simulink model "W08_F_mission"  (R2024b)
settings: Solver=ode4  StartTime=0  StopTime=T_final  FixedStep=h  RelTol=1e-3
values from neighbouring files (symbols this model uses):
  beta_c = pi/2    (= 1.57079632679)    [W08_0_setup.m]
  Delta = 5    [W08_0_setup.m]
  E_hold = 0    [W08_0_setup.m]
  e_min = 0.3    [W08_0_setup.m]
  h = 0.02    [W08_0_setup.m]    (also in W08_1_build_dp.m = add_line(sys, [a; via; b]))
  hand_over = 1    [W08_0_setup.m]
  k_neg = cfg.k_neg    [W08_0_setup.m]
  k_pos = cfg.k_pos    [W08_0_setup.m]
  Kd = 100    [W08_0_setup.m]
  Kd_x = 60    [W08_0_setup.m]
  Ki_x = 3    [W08_0_setup.m]
  Kp = 300    [W08_0_setup.m]
  Kp_x = 30    [W08_0_setup.m]
  mp = 25    [W08_0_setup.m]
  N_hold = 0    [W08_0_setup.m]
  N_max = min(2*cfg.y_pont*(cfg.k_pos*cfg.n_max^2 - X_max/2),              2*cfg.y_pont*(X_max/2 + cfg.k_neg*cfg.n_min^2))    [W08_0_setup.m]
  R_arrive = 2    [W08_0_setup.m]
  rp = [0.05 0 -0.35]'    [W08_0_setup.m]
  T_hold = 40    [W08_0_setup.m]
  T_max = cfg.k_pos*cfg.n_max^2    [W08_0_setup.m]
  T_min = -cfg.k_neg*cfg.n_min^2    [W08_0_setup.m]
  V_c = 0.3    [W08_0_setup.m]
  WP_E = [0  0 40]'    [W08_0_setup.m]
  WP_N = [0 40 40]'    [W08_0_setup.m]
  x0 = zeros(12,1)    [W08_0_setup.m]    (also in W08_E_cascade_gains.m = zeros(12,1);  x0(8) = 5)
  X_ff = 60    [W08_0_setup.m]
  X_max = 120    [W08_0_setup.m]
  y_pont = cfg.y_pont    [W08_0_setup.m]
settings Model: Creator=admin  LastModifiedBy=admin
settings DataIOCC: ReturnWorkspaceOutputs=off

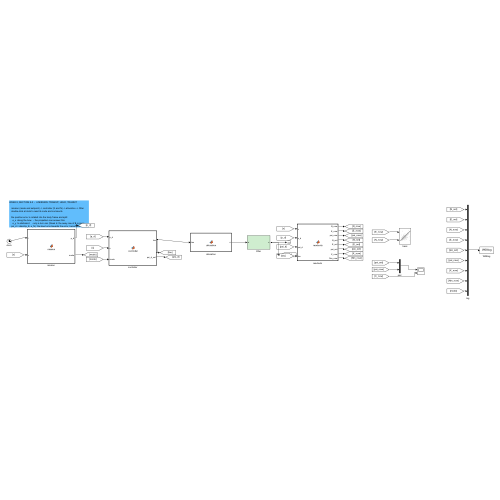
[thumbnail: Simulink's stored preview of the top-level diagram]
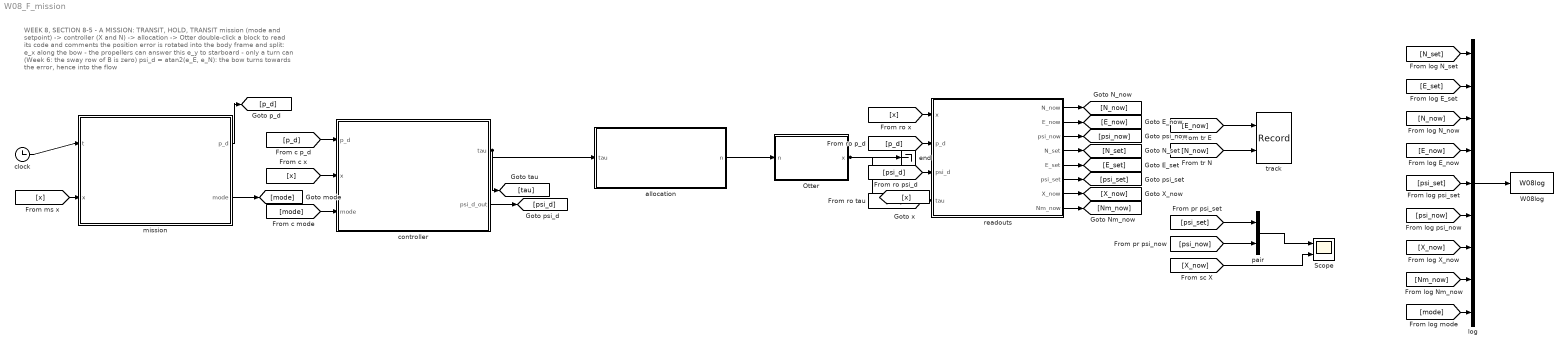
== system W08_F_mission ==
  note: WEEK 8, SECTION 8-5  -  A MISSION: TRANSIT, HOLD, TRANSIT
      |
      |    mission (mode and setpoint) -> controller (X and N) -> allocation -> Otter
      |    double-click a block to read its code and comments
      |
      |    the position error is rotated into the body frame and split:
      |      e_x  along the bow   - the propellers can answer this
      |      e_y  to starboard    - only a turn can (Week 6: the sway row of B is zero)
      |    psi_d = atan2(e_E, e_N): the bow turns towards the error, hence into the flow
  Otter : Subsystem
  Scope : Scope  NumInputPorts=2
  W08log : ToWorkspace  VariableName=W08log  SaveFormat=Structure With Time  SampleTime=-1
  allocation : MATLAB Function  TreatAsAtomicUnit=on
  clock : Clock
  controller : MATLAB Function  TreatAsAtomicUnit=on
  end : Terminator
  log : Mux  Inputs=9
  mission : MATLAB Function  TreatAsAtomicUnit=on
  pair : Mux  Inputs=2
  readouts : MATLAB Function  TreatAsAtomicUnit=on
  track : Record  FileSettingsInternal="{\"entries\":[{\"content\":{\"excelSettings\":{\"content\":{},\"type\":\"Streamout.ExcelSettings\"}},\"type\":\"Streamout.FileSettingStorage\",\"uuid\":\"\"}],\"packageUris\":[\"http:\\/\\/schema.mathworks.com\\/mf0\\/streamout_blocks\\/R2020a\"],\"version\":\"1.0\"}"  Layout=[1 1]  SignalsInternal="{\"entries\":[{\"content\":{\"signals\":[{\"content\":{\"blockPath\":[],\"dimensions\":[1],\"domain\":\"\",\"lineColor\":\"#a2142f\",\"plots\":[ 1 ],\"port\":1,\"signalID\":1,\"signalName\":\"XY Graph:1\"},\"type\":\"RecordBlkView.Signal\",\"uuid\":\"\"},{\"content\":{\"blockPath\":[],\"dimensions\":[1],\"domain\":\"\",\"lineColor\":\"#139fff\",\"plots\":[ 1 ],\"port\":2,\"signalID\":2,\"signalName\":\"XY Graph:2\"},\"type\":\"RecordBlkView.Signal\",\"uuid\":\"\"}]},\"type\":\"RecordBlkView.InputSignals\",\"uuid\":\"\"}],\"packageUris\":[\"http:\\/\\/schema.mathworks.com\\/mf0\\/streamout_blocks\\/R2020a\"],\"version\":\"1.0\"}"  VisualizationBindings="{\"xyplotplugin\":{\"info\":[{\"series\":[{\"bindingParametersList\":[{\"parameter\":\"X-Axis\",\"signalID\":1,\"signalName\":\"XY Graph:1\"},{\"parameter\":\"Y-Axis\",\"signalID\":2,\"signalName\":\"XY Graph:2\"}],\"seriesID\":0}],\"subplotID\":1}]}}"  CompatibilityTag=XY
  wires:
  clock/1 -> mission/1(t)
  [x] -> mission/2(x)
  mission/1(p_d) -> [p_d]
  mission/2(mode) -> [mode]
  [p_d] -> controller/1(p_d)
  [x] -> controller/2(x)
  [mode] -> controller/3(mode)
  controller/1(tau) -> [tau], allocation/1(tau)
  controller/2(psi_d_out) -> [psi_d]
  allocation/1(n) -> Otter/1(n)
  Otter/1(x) -> [x], end/1
  [x] -> readouts/1(x)
  [p_d] -> readouts/2(p_d)
  [psi_d] -> readouts/3(psi_d)
  [tau] -> readouts/4(tau)
  readouts/1(N_now) -> [N_now]
  readouts/2(E_now) -> [E_now]
  readouts/3(psi_now) -> [psi_now]
  readouts/4(N_set) -> [N_set]
  readouts/5(E_set) -> [E_set]
  readouts/6(psi_set) -> [psi_set]
  readouts/7(X_now) -> [X_now]
  readouts/8(Nm_now) -> [Nm_now]
  [E_now] -> track/1
  [N_now] -> track/2
  [psi_set] -> pair/1
  [psi_now] -> pair/2
  pair/1 -> Scope/1
  [X_now] -> Scope/2
  [N_set] -> log/1
  [E_set] -> log/2
  [N_now] -> log/3
  [E_now] -> log/4
  [psi_set] -> log/5
  [psi_now] -> log/6
  [X_now] -> log/7
  [Nm_now] -> log/8
  [mode] -> log/9
  log/1 -> W08log/1

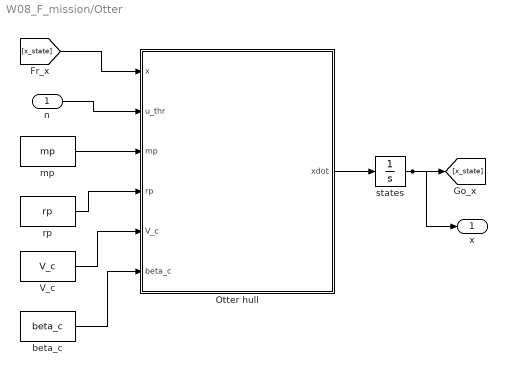
== system W08_F_mission/Otter ==
  n : Inport
  Otter hull : MATLAB Function  TreatAsAtomicUnit=on
  V_c : Constant  Value=V_c
  beta_c : Constant  Value=beta_c
  mp : Constant  Value=mp
  rp : Constant  Value=rp
  states : Integrator  InitialCondition=x0
  x : Outport
  wires:
  beta_c/1 -> Otter hull/6(beta_c)
  rp/1 -> Otter hull/4(rp)
  n/1 -> Otter hull/2(u_thr)
  [x_state] -> Otter hull/1(x)
  Otter hull/1(xdot) -> states/1
  mp/1 -> Otter hull/3(mp)
  V_c/1 -> Otter hull/5(V_c)
  states/1 -> [x_state], x/1

== matlab function W08_F_mission/controller ==
  settings: updateMethod=DISCRETE  sampleTime=h
  data: p_d input; tau output double size=[2 1]; x input; mode input; psi_d_out output; Kp_x parameter; Ki_x parameter; Kd_x parameter; e_min parameter; X_max parameter; Kp parameter; Kd parameter; N_max parameter; h parameter; X_ff parameter; Delta parameter; hand_over parameter
function [tau, psi_d_out] = controller(p_d, x, mode, Kp_x, Ki_x, Kd_x, e_min, X_max, Kp, Kd, N_max, h, X_ff, Delta, hand_over)
%#codegen
%  ────────────────────────────────────────────────────────────────────────
%  1) 얼마의 힘이 필요한가 — NED 에서 / how much force is needed, in NED
%
%     위치 오차에 대한 PID 를 **북·동 두 방향 모두**에 대해 쓴다. 나오는 것은
%     "이만큼의 힘이 이 방향으로 필요하다" 는 벡터 f 다. 아직 추진기 이야기가 아니다.
%     A PID on the position error, in both north and east: the result is a vector
%     saying how much force is wanted and in which direction. Not yet a thruster.
psi = x(12);  u = x(1);  v = x(2);  r = x(6);
e_n = p_d(1) - x(7);  e_e = p_d(2) - x(8);
v_n = u*cos(psi) - v*sin(psi);        % 속도를 NED 로 / the velocity in NED
v_e = u*sin(psi) + v*cos(psi);
persistent In Ie
if isempty(In), In = 0;  Ie = 0; end
f_n = Kp_x*e_n + In - Kd_x*v_n;
f_e = Kp_x*e_e + Ie - Kd_x*v_e;
%  ────────────────────────────────────────────────────────────────────────
%  2) 그 힘의 방향으로 뱃머리를 / point the bow along that force
%
%     이 선체가 낼 수 있는 힘은 **뱃머리 방향뿐**이다 (6주차 §6-3: B 의 둘째 행이 0).
%     그러므로 필요한 힘 f 를 내려면 뱃머리가 f 를 향해야 한다.
%     조류가 밀면 적분이 상류 쪽 힘을 배우고, 뱃머리는 그것을 따라 조류에 맞선다.
%     The only force this hull can make points along its bow (Week 6 §6-3), so to
%     deliver f the bow must point along f. Under a current the integral learns an
%     upstream force, and the bow follows it into the flow.
f  = hypot(f_n, f_e);
persistent psi_last
if isempty(psi_last), psi_last = psi; end
if f > e_min, psi_last = atan2(f_e, f_n); end   % 힘이 작으면 방향이 뜻을 잃는다 / too small to point by
psi_d = psi_last;
%  ────────────────────────────────────────────────────────────────────────
%  2b) 이동 중이면 목표를 향해 / in transit, point at the waypoint
if mode == 1, psi_d = atan2(e_e, e_n); end
%  ────────────────────────────────────────────────────────────────────────
%  3) 뱃머리 방향의 성분만 추진기로 / only the along-bow part reaches the propellers
%     X = f 를 뱃머리에 정사영한 것. 옆 성분 f_y 는 아무도 낼 수 없다 —
%     그것이 이 주차가 재는 양이다.
%     X is f projected on the bow; the part across it, f_y, nobody can make.
X = f_n*cos(psi) + f_e*sin(psi);
if mode == 1
    X = X_ff;                                  % 이동 중에는 일정한 추진력 / a constant push
    if hand_over ~= 0, In = 0;  Ie = 0; end    % 유지를 깨끗한 적분으로 시작 / a clean integral for the hold
end
X = min(max(X, -X_max), X_max);
%  적분은 힘이 한계에 있지 않을 때만 쌓는다 (2주차 §2-11) / integrate only while there is room
if abs(X) < X_max - 1e-9
    In = In + h*Ki_x*e_n;
    Ie = Ie + h*Ki_x*e_e;
end
%  ────────────────────────────────────────────────────────────────────────
%  4) 요 모멘트: 4주차의 오토파일럿 그대로 / the yaw moment: the Week 4 autopilot
ee = atan2(sin(psi_d - psi), cos(psi_d - psi));
N  = Kp*ee - Kd*r;
N  = min(max(N, -N_max), N_max);
if mode == 3, X = 0;  N = 0; end                % 끝 / done
tau = [X; N];
psi_d_out = psi_d;

== matlab function W08_F_mission/mission ==
  settings: updateMethod=DISCRETE  sampleTime=h
  data: t input; p_d output double size=[2 1]; x input; mode output; N_hold parameter; E_hold parameter; WP_N parameter; WP_E parameter; R_arrive parameter; T_hold parameter; h parameter
function [p_d, mode] = mission(t, x, N_hold, E_hold, WP_N, WP_E, R_arrive, T_hold, h)
%#codegen
%  임무 논리: 이동(1) -> 유지(2) -> 다음 지점 -> ... -> 끝(3)
%  The mission: transit (1) -> hold (2) -> the next waypoint -> ... -> done (3)
%
%  상태를 가진 블록이므로 이산 실행이다 (set_mlfcn 의 h). 규칙은 두 줄뿐이다:
%    이동 중이고 목표에 R_arrive 안으로 들어오면 유지로 바꾸고 시계를 0 으로.
%    유지 중이고 T_hold 가 지나면 다음 지점으로 가며 이동으로 바꾼다.
%  A block with memory, so it runs at a fixed rate. Two rules only:
%    in transit and inside R_arrive  -> hold, and reset the clock
%    in hold and T_hold has passed   -> the next waypoint, and transit
persistent k mode_ held
if isempty(k), k = 1; mode_ = 1; held = 0; end
d = hypot(WP_N(k) - x(7), WP_E(k) - x(8));
if mode_ == 1 && d < R_arrive
    mode_ = 2;  held = 0;
elseif mode_ == 2
    held = held + h;
    if held >= T_hold
        if k < numel(WP_N), k = k + 1;  mode_ = 1;  else, mode_ = 3; end
    end
end
p_d  = [WP_N(k); WP_E(k)];
mode = mode_;

== matlab function W08_F_mission/allocation ==
  data: tau input; n output double size=[2 1]; y_pont parameter; k_pos parameter; k_neg parameter; T_max parameter; T_min parameter
function n = allocation(tau, y_pont, k_pos, k_neg, T_max, T_min)
%#codegen
%  6주차의 배분 그대로. 이번에는 X 가 상수가 아니라 위치 루프의 출력이다.
%  The allocation of Week 6, with X now coming from the position loop.
T1 = tau(1)/2 + tau(2)/(2*y_pont);
T2 = tau(1)/2 - tau(2)/(2*y_pont);
s = 1;
if T1 > T_max, s = min(s, T_max/T1); end
if T2 > T_max, s = min(s, T_max/T2); end
if T1 < T_min, s = min(s, T_min/T1); end
if T2 < T_min, s = min(s, T_min/T2); end
T1 = s*T1;  T2 = s*T2;
k1 = k_pos;  if T1 < 0, k1 = k_neg; end
k2 = k_pos;  if T2 < 0, k2 = k_neg; end
n = [sign(T1)*sqrt(abs(T1)/k1); sign(T2)*sqrt(abs(T2)/k2)];

== matlab function W08_F_mission/Otter/Otter hull ==
  data: x input; xdot output double size=[12 1]; u_thr input; mp input; rp input; V_c input; beta_c input
function xdot = otter_hull(x, u_thr, mp, rp, V_c, beta_c)
% Fossen's otter.m, called unchanged from Tools/MSS/VESSELS.
%
%   x       12 states, fed back from the integrator
%   u_thr   propeller shaft speeds [rad/s]
%
% otter.m is not written for code generation, so the call is extrinsic and
% xdot has to be pre-sized for Simulink to know the output width.
coder.extrinsic('otter');

xdot = zeros(12,1);
xdot = otter(x, u_thr, mp, rp, V_c, beta_c);
end

== matlab function W08_F_mission/readouts ==
  data: x input; N_now output double size=[1 1]; p_d input; psi_d input; tau input; E_now output; psi_now output; N_set output; E_set output; psi_set output; X_now output; Nm_now output
function [N_now, E_now, psi_now, N_set, E_set, psi_set, X_now, Nm_now] = readouts(x, p_d, psi_d, tau)
%#codegen
%  표시와 기록만 한다 / display and logging only
N_now = x(7);  E_now = x(8);  psi_now = x(12)*180/pi;
N_set = p_d(1);  E_set = p_d(2);  psi_set = psi_d*180/pi;
X_now = tau(1);  Nm_now = tau(2);
